simulink model "both_on_off"  (R2015b)
settings: Solver=ode23tb  StartTime=0.0  StopTime=2  RelTol=1e-3
PreLoadFcn:
  | load  power_3levelVSC.mat
  | Ts_Power=5e-6;
  | Ts_Control=100e-6;
libraries: powerlib x29, powerlib_extras x7, powerlib_meascontrol x6, simulink x3
settings Model: Creator=Pouyan  LastModifiedBy=fujitsu
settings DataIOCC: SaveFormat=Array  SignalLoggingSaveFormat=ModelDataLogs
settings OptimizationCC: ExpressionDepthLimit=2147483647
settings DebuggingCC: UnderspecifiedInitializationDetection=Classic  MergeDetectMultiDrivingBlocksExec=none  SolverPrmCheckMsg=warning  FcnCallInpInsideContextMsg=UseLocalSettings  StateNameClashWarn=warning
settings HardwareCC: ProdBitPerPointer=32  ProdLargestAtomicFloat=None  ProdIntDivRoundTo=Undefined  ProdEndianess=Unspecified  ProdWordSize=32  ProdHWDeviceType=32-bit Generic
settings GRTTargetCC: GeneratePreprocessorConditionals=Disable all  CombineOutputUpdateFcns=off  GRTInterface=on
settings ConfigComp: CovModelRefEnable=Off

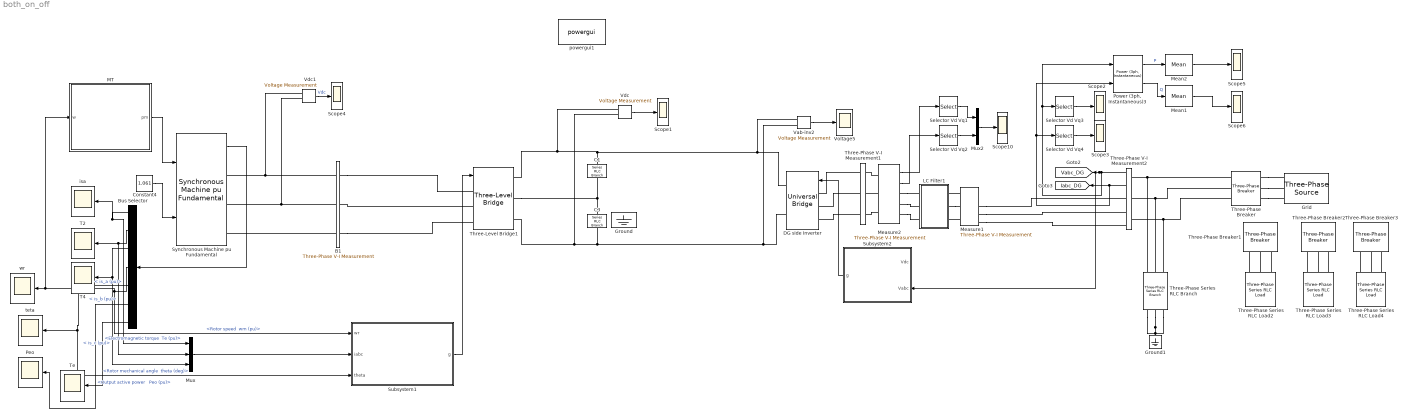
== system both_on_off ==
  B1 : powerlib/Measurements/Three-Phase V-I Measurement  VoltageMeasurement=phase-to-ground  SetLabelV=on  LabelV=Vabc_B1  Vpu=off  VpuLL=off  CurrentMeasurement=yes  SetLabelI=on  LabelI=Iabc_B1  Ipu=off  Pbase=100e6  Vbase=500e3  OutputType=Magnitude  PhasorSimulation=off  PSBequivalent=0
  Bus Selector : BusSelector  OutputSignals="Stator current. is_a (pu),Stator current. is_b (pu),Stator current. is_c (pu),Mechanical.Rotor speed  wm (pu),Mechanical.Rotor mechanical angle  theta (deg),Output active power   Peo (pu),Mechanical.Electromagnetic torque  Te (pu)"
  C1 : powerlib/Elements/Series RLC Branch  LConnTagsString=__new0  RConnTagsString=__new0  BranchType=C  Resistance=1.0  Inductance=1.0  SetiL0=off  InitialCurrent=0  Capacitance=75000e-06  Setx0=off  InitialVoltage=0  Measurements=None
  C3 : powerlib/Elements/Series RLC Branch  LConnTagsString=__new0  RConnTagsString=__new0  BranchType=C  Resistance=1.0  Inductance=1.0  SetiL0=off  InitialCurrent=0  Capacitance=75000e-06  Setx0=off  InitialVoltage=0  Measurements=None
  Constant4 : Constant  Value=1.061
  DG side Inverter : powerlib/Power Electronics/Universal Bridge  Arms=3  SnubberResistance=10000  SnubberCapacitance=inf  Device=IGBT / Diodes  Ron=1e-4  Lon=0  ForwardVoltages="[  1  1  ]"  ForwardVoltage=.8  GTOparameters=[ 10e-6 , 20e-6 ]  IGBTparameters=[ 1e-6 , 2e-6 ]  Measurements=None  Measurements_2=None  converterType=Rectifier
  Grid : powerlib/Electrical Sources/Three-Phase Source  InternalConnection=Yg  VoltagePhases=off  Voltage=400  PhaseAngle=0  Voltage_phases=[25e3 25e3 25e3]/sqrt(3)  PhaseAngles_phases=[0 -120 +120]  Frequency=50  NonIdealSource=on  SpecifyImpedance=off  Resistance=0.02  Inductance=0.3e-3  ShortCircuitLevel=100e6  BaseVoltage=25e3  XRratio=7  BusType=swing  Pref=0  Qref=0  Prefabc=[10e3, 10e3, 10e3]  Qrefabc=[0, 0, 0]  Qmin=-inf  Qmax=inf
  Ground : powerlib/Elements/Ground  LConnTagsString=a
  Ground1 : powerlib/Elements/Ground  LConnTagsString=a
  LC Filter1 : Subsystem
  MT : Subsystem
  Mean1 : powerlib_meascontrol/Measurements/Mean  Freq=50  Vinit=0  Ts=50e-6
  Mean2 : powerlib_meascontrol/Measurements/Mean  Freq=50  Vinit=0  Ts=50e-6
  Measure1 : powerlib/Measurements/Three-Phase V-I Measurement  VoltageMeasurement=phase-to-phase  SetLabelV=off  LabelV=V1  Vpu=off  VpuLL=off  CurrentMeasurement=yes  SetLabelI=off  LabelI=I1  Ipu=off  Pbase=10e3  Vbase=400  OutputType=Magnitude  PhasorSimulation=off  PSBequivalent=0
  Measure2 : powerlib/Measurements/Three-Phase V-I Measurement  VoltageMeasurement=phase-to-phase  SetLabelV=off  LabelV=V1  Vpu=off  VpuLL=on  CurrentMeasurement=yes  SetLabelI=off  LabelI=I1  Ipu=on  Pbase=30e3  Vbase=380  OutputType=Magnitude  PhasorSimulation=off  PSBequivalent=0
  Mux : Mux  Inputs=3
  Mux2 : Mux  Inputs=2
  Peo : Scope
  "Power (3ph, Instantaneous)3" : powerlib_meascontrol/Measurements/Power (3ph, Instantaneous)
  Scope{1..6,10} (7 alike) : Scope
  Selector Vd Vq{1..4} (4 alike) : Selector  InputPortWidth=3  IndexOptions=Index vector (dialog)  Indices=[1]  OutputSizes=1
  Subsystem1 : Subsystem  mask{kp=1, ki=5}
  Subsystem2 : Subsystem  mask{kp=0.0001, ki=5}
  Synchronous Machine pu Fundamental : powerlib/Machines/Synchronous Machine pu Fundamental  PresetModel=No  MechanicalLoad=Mechanical power Pm  ShowDetailedParameters=on  RotorType=Salient-pole  Units=per unit fundamental parameters  MeasurementBus=off  NominalParameters="[ 60e3  500 1600]"  Stator="[ 0.2503  0.114  0.6875  0.6875 ]"  Field="[ 1  10e15/(100*pi)]"  Dampers2=[0.0652, 0.5134, 0.0287, 0.2553, 7.765e-3, 0.9167 ]  Dampers1="[ 1.17E-02  0.182  1.97E-02  0.384 ]"  Mechanical=[ 6 0 2]  PolePairs=20  InitialConditions="[ 0  0  0  0  0  0  0  0  1 ]"  SetSaturation=off  Saturation=[0.6404,0.7127,0.8441,0.9214,0.9956,1.082,1.19,1.316,1.457;0.7,0.7698,0.8872,0.9466,0.9969,1.046,1.1,1.151,1.201]  LoadFlowParameters=[1,0,0,0,0]  TsPowergui=0  TsBlock=-1  IterativeModel=Trapezoidal non iterative  BusType=swing  Pref=0  Qref=0  Qmin=-inf  Qmax=inf  PLF=0  QLF=0
  T2 : Scope
  T4 : Scope
  Te : Scope
  Three-Level Bridge1 : powerlib/Power Electronics/Three-Level Bridge  Arms=3  SnubberResistance=100  SbubberCapacitance=1e-6  Device=IGBT / Diodes  Ron=5e-3  ForwardVoltages=[370 1]  Measurements=All voltages and currents
  Three-Phase Series RLC Branch : powerlib/Elements/Three-Phase Series RLC Branch  LConnTagsString=A|B|C  RConnTagsString=A|B|C  BranchType=R  Resistance=400^2/50000  Inductance=1e-3  Capacitance=1e-6  Measurements=None
  Three-Phase Series RLC Load2 : powerlib/Elements/Three-Phase Series RLC Load  LConnTagsString=A|B|C  Configuration=Y (grounded)  NominalVoltage=380  Vabc=[1e3 1e3 1e3]  Vabcp=[1e3 1e3 1e3]  NominalFrequency=50  UnbalancedPower=off  ActivePower=50e3  InductivePower=0  CapacitivePower=0  Pabc=[10e3 9e3 11e3]  QLabc=[100 90 110]  QCabc=[100 90 110]  Pabcp=[10e3 9e3 11e3]  QLabcp=[100 90 110]  QCabcp=[100 90 110]  Measurements=None  LoadType=constant Z
  Three-Phase Series RLC Load3 : powerlib/Elements/Three-Phase Series RLC Load  LConnTagsString=A|B|C  Configuration=Y (grounded)  NominalVoltage=380  Vabc=[1e3 1e3 1e3]  Vabcp=[1e3 1e3 1e3]  NominalFrequency=50  UnbalancedPower=off  ActivePower=15e3  InductivePower=0  CapacitivePower=0  Pabc=[10e3 9e3 11e3]  QLabc=[100 90 110]  QCabc=[100 90 110]  Pabcp=[10e3 9e3 11e3]  QLabcp=[100 90 110]  QCabcp=[100 90 110]  Measurements=None  LoadType=constant Z
  Three-Phase Series RLC Load4 : powerlib/Elements/Three-Phase Series RLC Load  LConnTagsString=A|B|C  Configuration=Y (grounded)  NominalVoltage=380  Vabc=[1e3 1e3 1e3]  Vabcp=[1e3 1e3 1e3]  NominalFrequency=50  UnbalancedPower=off  ActivePower=30e3  InductivePower=0  CapacitivePower=0  Pabc=[10e3 9e3 11e3]  QLabc=[100 90 110]  QCabc=[100 90 110]  Pabcp=[10e3 9e3 11e3]  QLabcp=[100 90 110]  QCabcp=[100 90 110]  Measurements=None  LoadType=constant Z
  Three-Phase V-I Measurement1 : powerlib/Measurements/Three-Phase V-I Measurement  VoltageMeasurement=no  SetLabelV=off  LabelV=Vabc  Vpu=on  VpuLL=off  CurrentMeasurement=no  SetLabelI=off  LabelI=Iabc  Ipu=on  Pbase=300e3  Vbase=208  OutputType=Complex  PhasorSimulation=off  PSBequivalent=0
  Three-Phase V-I Measurement2 : powerlib/Measurements/Three-Phase V-I Measurement  VoltageMeasurement=phase-to-phase  SetLabelV=off  LabelV=Vabc  Vpu=off  VpuLL=on  CurrentMeasurement=yes  SetLabelI=off  LabelI=Iabc  Ipu=on  Pbase=50e3  Vbase=400  OutputType=Complex  PhasorSimulation=off  PSBequivalent=0
  Three-Phase Breaker : powerlib/Elements/Three-Phase Breaker  InitialState=closed  SwitchA=on  SwitchB=on  SwitchC=on  SwitchTimes=[1]  External=off  BreakerResistance=0.01  SnubberResistance=1e6  SnubberCapacitance=inf  Measurements=None
  Three-Phase Breaker1 : powerlib/Elements/Three-Phase Breaker  InitialState=open  SwitchA=on  SwitchB=on  SwitchC=on  SwitchTimes=[8]  External=off  BreakerResistance=0.01  SnubberResistance=1e6  SnubberCapacitance=inf  Measurements=None
  Three-Phase Breaker2 : powerlib/Elements/Three-Phase Breaker  InitialState=closed  SwitchA=on  SwitchB=on  SwitchC=on  SwitchTimes=[6 9]  External=off  BreakerResistance=0.01  SnubberResistance=1e6  SnubberCapacitance=inf  Measurements=None
  Three-Phase Breaker3 : powerlib/Elements/Three-Phase Breaker  InitialState=open  SwitchA=on  SwitchB=on  SwitchC=on  SwitchTimes=[4]  External=off  BreakerResistance=0.01  SnubberResistance=1e6  SnubberCapacitance=inf  Measurements=None
  Vab-inv2 : powerlib/Measurements/Voltage Measurement  Tag=PoWeRsYsTeMmEaSuReMeNt  PhasorSimulation=off  OutputType=Magnitude  PSBequivalent=0
  "Vdc " : powerlib/Measurements/Voltage Measurement  Tag=PoWeRsYsTeMmEaSuReMeNt  PhasorSimulation=off  OutputType=Magnitude  PSBequivalent=0
  Vdc1 : powerlib/Measurements/Voltage Measurement  Tag=PoWeRsYsTeMmEaSuReMeNt  PhasorSimulation=off  OutputType=Magnitude  PSBequivalent=0
  Voltage5 : Scope
  isa : Scope
  powergui1 : powerlib/powergui  Priority=2  SimulationMode=Discrete  SolverType=Tustin/Backward Euler (TBE)  SampleTime=Ts_Power  frequency=60  SPID=off  DisableSnubberDevices=off  DisableRonSwitches=off  DisableVfSwitches=off  SwTol=0  DisplayEquations=off  Interpol=off  ExternalGateDelay=off  methode=off  Ts=0  FunctionMessages=off  echomessages=off  HookPort=off  EnableUseOfTLC=off  x0status=blocks  frequencyindice=0  Pbase=100e6  ErrMax=1e-4  Iterations=50  UnitsV=kV  UnitsW=MW  buscounter=0  RestoreLinks=warning  ResistiveCurrentMeasurement=off  Frange=logspace(0,3,50)  Ylog=off  Xlog=off  ShowGrid=off  save=off  variable=ZData  structure=VaIa  ZoomFFT=on  StartTime=0.2  cycles=2  DisplayStyle=1  fundamental=60  FreqAxis=off  MaxFrequency=1000  frequencyindicesteady=1  RmsSteady=2  display=off
  teta : Scope
  wr : Scope
  tag scope: Iabc_DG=global, Vabc_DG=global
  wires:
  "Vdc "/1 -> Scope1/1
  MT/1(pm) -> Synchronous Machine pu Fundamental/1
  Synchronous Machine pu Fundamental/1 -> Bus Selector/1
  Bus Selector/4 -> Subsystem1/1(wr), MT/1(w), wr/1  "<Rotor speed  wm (pu)>"
  Constant4/1 -> Synchronous Machine pu Fundamental/2
  Vdc1/1 -> Scope4/1  "Vdc"
  Bus Selector/1 -> Mux/1, isa/1  "< is_a (pu)>"
  Bus Selector/2 -> T2/1, Mux/2  "< is_b (pu)>"
  Bus Selector/3 -> Mux/3, T4/1  "< is_c (pu)>"
  Bus Selector/5 -> Subsystem1/3(theta), teta/1  "<Rotor mechanical angle  theta (deg)>"
  Mux/1 -> Subsystem1/2(iabc)
  Subsystem1/1(g) -> Three-Level Bridge1/1
  Three-Phase V-I Measurement2/1 -> Subsystem2/2(Vabc), [Vabc_DG], "Power (3ph, Instantaneous)3"/1, Selector Vd Vq3/1
  Three-Phase V-I Measurement2/2 -> "Power (3ph, Instantaneous)3"/2, Selector Vd Vq4/1, [Iabc_DG]
  Vab-inv2/1 -> Voltage5/1
  Mux2/1 -> Scope10/1
  Selector Vd Vq1/1 -> Mux2/1
  Selector Vd Vq2/1 -> Mux2/2
  Measure2/1 -> Selector Vd Vq1/1
  Measure2/2 -> Selector Vd Vq2/1
  Selector Vd Vq3/1 -> Scope2/1
  Selector Vd Vq4/1 -> Scope3/1
  "Power (3ph, Instantaneous)3"/1 -> Mean2/1  "P"
  "Power (3ph, Instantaneous)3"/2 -> Mean1/1  "Q"
  Mean2/1 -> Scope5/1
  Mean1/1 -> Scope6/1
  Subsystem2/1(g) -> DG side Inverter/1
  Bus Selector/6 -> Peo/1  "<Output active power   Peo (pu)>"
  Bus Selector/7 -> Te/1  "<Electromagnetic torque  Te (pu)>"
  connections:
  C3/LConn1 -- C1/RConn1 -- Three-Level Bridge1/RConn2
  DG side Inverter/RConn2 -- Vab-inv2/LConn2 -- Three-Level Bridge1/RConn3 -- "Vdc "/LConn2 -- C3/RConn1
  Vab-inv2/LConn1 -- DG side Inverter/RConn1 -- C1/LConn1 -- Three-Level Bridge1/RConn1 -- "Vdc "/LConn1
  B1/RConn1 -- Three-Level Bridge1/LConn1
  B1/RConn3 -- Three-Level Bridge1/LConn3
  Three-Level Bridge1/LConn2 -- B1/RConn2
  B1/LConn1 -- Vdc1/LConn1 -- Synchronous Machine pu Fundamental/RConn1
  B1/LConn2 -- Vdc1/LConn2 -- Synchronous Machine pu Fundamental/RConn2
  B1/LConn3 -- Synchronous Machine pu Fundamental/RConn3
  Three-Phase Breaker/LConn1 -- Three-Phase Series RLC Branch/LConn1 -- Three-Phase V-I Measurement2/LConn1
  Three-Phase Series RLC Branch/LConn2 -- Three-Phase Breaker/LConn2 -- Three-Phase V-I Measurement2/LConn2
  Three-Phase Series RLC Branch/LConn3 -- Three-Phase Breaker/LConn3 -- Three-Phase V-I Measurement2/LConn3
  Measure1/RConn2 -- Three-Phase V-I Measurement2/RConn2
  Measure1/RConn3 -- Three-Phase V-I Measurement2/RConn3
  Measure1/RConn1 -- Three-Phase V-I Measurement2/RConn1
  Three-Phase V-I Measurement1/RConn1 -- DG side Inverter/LConn1
  Three-Phase V-I Measurement1/RConn2 -- DG side Inverter/LConn2
  Three-Phase V-I Measurement1/RConn3 -- DG side Inverter/LConn3
  Measure1/LConn1 -- LC Filter1/RConn1
  Measure1/LConn3 -- LC Filter1/RConn3
  Measure2/LConn2 -- Three-Phase V-I Measurement1/LConn2
  Measure2/LConn1 -- Three-Phase V-I Measurement1/LConn1
  Measure2/LConn3 -- Three-Phase V-I Measurement1/LConn3
  Measure2/RConn1 -- LC Filter1/LConn1
  Measure2/RConn2 -- LC Filter1/LConn2
  Measure2/RConn3 -- LC Filter1/LConn3
  LC Filter1/RConn2 -- Measure1/LConn2
  Three-Phase Breaker/RConn1 -- Grid/RConn1
  Three-Phase Breaker/RConn2 -- Grid/RConn2
  Three-Phase Breaker/RConn3 -- Grid/RConn3
  Three-Phase Series RLC Load2/LConn1 -- Three-Phase Breaker1/RConn3
  Three-Phase Series RLC Load2/LConn2 -- Three-Phase Breaker1/RConn2
  Three-Phase Series RLC Load2/LConn3 -- Three-Phase Breaker1/RConn1
  Three-Phase Series RLC Load3/LConn1 -- Three-Phase Breaker2/RConn3
  Three-Phase Series RLC Load3/LConn2 -- Three-Phase Breaker2/RConn2
  Three-Phase Series RLC Load3/LConn3 -- Three-Phase Breaker2/RConn1
  Three-Phase Series RLC Load4/LConn1 -- Three-Phase Breaker3/RConn3
  Three-Phase Series RLC Load4/LConn2 -- Three-Phase Breaker3/RConn2
  Three-Phase Series RLC Load4/LConn3 -- Three-Phase Breaker3/RConn1
  Three-Phase Series RLC Branch/RConn1 -- Three-Phase Series RLC Branch/RConn3 -- Three-Phase Series RLC Branch/RConn2 -- Ground1/LConn1

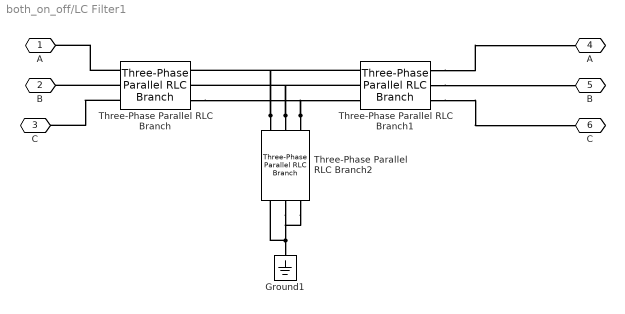
== system both_on_off/LC Filter1 ==
  Ground1 : powerlib/Elements/Ground  LConnTagsString=a
  Three-Phase Parallel RLC Branch : powerlib/Elements/Three-Phase Parallel RLC Branch  LConnTagsString=A|B|C  RConnTagsString=A|B|C  BranchType=L  Resistance=1  Inductance=5.7e-3  Capacitance=1e-6  Measurements=None
  Three-Phase Parallel RLC Branch1 : powerlib/Elements/Three-Phase Parallel RLC Branch  LConnTagsString=A|B|C  RConnTagsString=A|B|C  BranchType=R  Resistance=0.00001  Inductance=5.7e-3  Capacitance=1e-6  Measurements=None
  Three-Phase Parallel RLC Branch2 : powerlib/Elements/Three-Phase Parallel RLC Branch  LConnTagsString=A|B|C  RConnTagsString=A|B|C  BranchType=C  Resistance=1  Inductance=5.7e-3  Capacitance=1000e-6  Measurements=None
  A : PMIOPort  Port=1  Side=Left
  B : PMIOPort  Port=2  Side=Left
  C : PMIOPort  Port=3  Side=Left
  "A " : PMIOPort  Port=4  Side=Right
  "B " : PMIOPort  Port=5  Side=Right
  "C " : PMIOPort  Port=6  Side=Right
  connections:
  Ground1/LConn1 -- Three-Phase Parallel RLC Branch2/RConn2 -- Three-Phase Parallel RLC Branch2/RConn1 -- Three-Phase Parallel RLC Branch2/RConn3
  Three-Phase Parallel RLC Branch1/RConn3 -- "C "/RConn1
  Three-Phase Parallel RLC Branch1/RConn2 -- "B "/RConn1
  Three-Phase Parallel RLC Branch1/RConn1 -- "A "/RConn1
  Three-Phase Parallel RLC Branch2/LConn3 -- Three-Phase Parallel RLC Branch1/LConn3 -- Three-Phase Parallel RLC Branch/RConn3
  Three-Phase Parallel RLC Branch2/LConn2 -- Three-Phase Parallel RLC Branch/RConn2 -- Three-Phase Parallel RLC Branch1/LConn2
  Three-Phase Parallel RLC Branch2/LConn1 -- Three-Phase Parallel RLC Branch/RConn1 -- Three-Phase Parallel RLC Branch1/LConn1
  Three-Phase Parallel RLC Branch/LConn3 -- C/RConn1
  Three-Phase Parallel RLC Branch/LConn2 -- B/RConn1
  Three-Phase Parallel RLC Branch/LConn1 -- A/RConn1

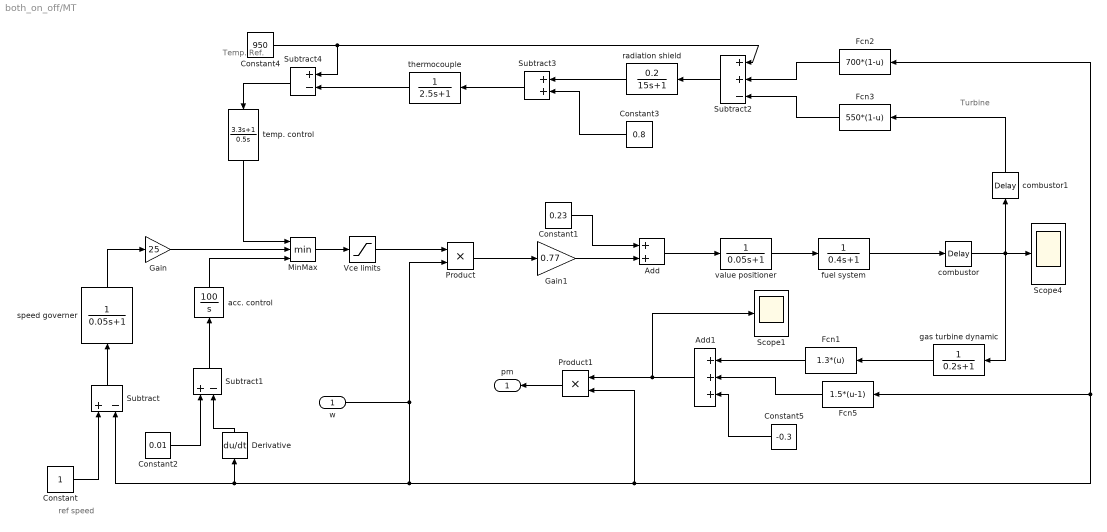
== system both_on_off/MT ==
  note: ref speed
  note: Temp.
      | Ref.
  note: Turbine
  w : Inport
  Add : Sum
  Add1 : Sum  Inputs=+++
  Constant : Constant
  Constant1 : Constant  Value=0.23
  Constant2 : Constant  Value=0.01
  Constant3 : Constant  Value=0.8
  Constant4 : Constant  Value=950
  Constant5 : Constant  Value=-0.3
  Derivative : Derivative  CoefficientInTFapproximation=0.001
  Fcn1 : Fcn  Expr=1.3*(u)
  Fcn2 : Fcn  Expr=700*(1-u)
  Fcn3 : Fcn  Expr=550*(1-u)
  Fcn5 : Fcn  Expr=1.5*(u-1)
  Gain : Gain  Gain=25
  Gain1 : Gain  Gain=0.77
  MinMax : MinMax  Inputs=3
  Product : Product  RndMeth=Zero
  Product1 : Product  RndMeth=Zero
  Scope1 : Scope
  Scope4 : Scope
  Subtract : Sum  Inputs=+-
  Subtract1 : Sum  Inputs=+-
  Subtract2 : Sum  Inputs=++-
  Subtract3 : Sum
  Subtract4 : Sum  Inputs=+-
  Vce limits : Saturate  UpperLimit=1.5  LowerLimit=-0.1
  acc. control : TransferFcn  Numerator=[0 100]  Denominator=[1 0]
  combustor : TransportDelay  DelayTime=0.01
  combustor1 : TransportDelay  DelayTime=0.04
  fuel system : TransferFcn  Denominator=[0.4 1]
  gas turbine dynamic : TransferFcn  Denominator=[0.2 1]
  radiation shield : TransferFcn  Numerator=[0.2]  Denominator=[15 1]
  speed governer : TransferFcn  Numerator=[0 1]  Denominator=[0.05 1]
  temp. control : TransferFcn  Numerator=[3.3 1]  Denominator=[0.5 0]
  thermocouple : TransferFcn  Denominator=[2.5 1]
  value positioner : TransferFcn  Denominator=[0.05 1]
  pm : Outport
  wires:
  Constant/1 -> Subtract/1
  Subtract/1 -> speed governer/1
  Vce limits/1 -> Product/1
  Product/1 -> Gain1/1
  Gain1/1 -> Add/2
  Constant1/1 -> Add/1
  Add/1 -> value positioner/1
  value positioner/1 -> fuel system/1
  fuel system/1 -> combustor/1
  combustor/1 -> gas turbine dynamic/1, combustor1/1, Scope4/1
  Add1/1 -> Scope1/1, Product1/1
  Gain/1 -> MinMax/2
  Derivative/1 -> Subtract1/2
  Constant2/1 -> Subtract1/1
  Subtract1/1 -> acc. control/1
  acc. control/1 -> MinMax/3
  MinMax/1 -> Vce limits/1
  combustor1/1 -> Fcn3/1
  Fcn3/1 -> Subtract2/3
  Fcn2/1 -> Subtract2/2
  radiation shield/1 -> Subtract3/1
  Constant3/1 -> Subtract3/2
  Subtract2/1 -> radiation shield/1
  Subtract3/1 -> thermocouple/1
  thermocouple/1 -> Subtract4/2
  Constant4/1 -> Subtract4/1, Subtract2/1
  Subtract4/1 -> temp. control/1
  temp. control/1 -> MinMax/1
  speed governer/1 -> Gain/1
  w/1 -> Product/2, Product1/2, Fcn2/1, Fcn5/1, Derivative/1, Subtract/2
  gas turbine dynamic/1 -> Fcn1/1
  Fcn1/1 -> Add1/1
  Constant5/1 -> Add1/3
  Fcn5/1 -> Add1/2
  Product1/1 -> pm/1

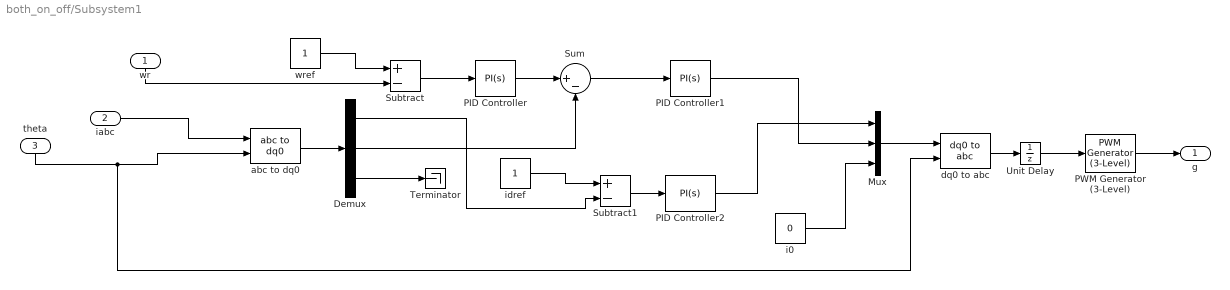
== system both_on_off/Subsystem1 ==
  wr : Inport
  iabc : Inport  Port=2
  theta : Inport  Port=3
  Demux : Demux  Outputs=3
  Mux : Mux  Inputs=3
  PID Controller : simulink/Continuous/PID Controller  Controller=PI  TimeDomain=Continuous-time  SampleTime=-1  IntegratorMethod=Forward Euler  FilterMethod=Forward Euler  Form=Parallel  UseFilter=on  ControllerParametersSource=internal  P=kp  I=ki  D=0  N=100  InitialConditionSource=internal  InitialConditionForIntegrator=0  InitialConditionForFilter=0  ExternalReset=none  LimitOutput=off  UpperSaturationLimit=inf  LowerSaturationLimit=-inf  LinearizeAsGain=on  AntiWindupMode=none  Kb=1  TrackingMode=off  Kt=1  PParamMin=[]  PParamMax=[]  IParamMin=[]  IParamMax=[]  DParamMin=[]  DParamMax=[]  NParamMin=[]  NParamMax=[]  KbParamMin=[]  KbParamMax=[]  KtParamMin=[]  KtParamMax=[]  POutMin=[]  POutMax=[]  IOutMin=[]  IOutMax=[]  DOutMin=[]  DOutMax=[]  NOutMin=[]  NOutMax=[]  KbOutMin=[]  KbOutMax=[]  KtOutMin=[]  KtOutMax=[]  IntegratorOutMin=[]  IntegratorOutMax=[]  FilterOutMin=[]  FilterOutMax=[]  SumOutMin=[]  SumOutMax=[]  SumI1OutMin=[]  SumI1OutMax=[]  SumI2OutMin=[]  SumI2OutMax=[]  SumI3OutMin=[]  SumI3OutMax=[]  SumDOutMin=[]  SumDOutMax=[]  SaturationOutMin=[]  SaturationOutMax=[]  IntegratorContinuousStateAttributes=''  IntegratorStateMustResolveToSignalObject=off  IntegratorRTWStateStorageClass=Auto  FilterContinuousStateAttributes=''  FilterStateMustResolveToSignalObject=off  FilterRTWStateStorageClass=Auto  DifferentiatorICPrevScaledInput=0  DifferentiatorOutMin=[]  DifferentiatorOutMax=[]
  PID Controller1 : simulink/Continuous/PID Controller  Controller=PI  TimeDomain=Continuous-time  SampleTime=-1  IntegratorMethod=Forward Euler  FilterMethod=Forward Euler  Form=Parallel  UseFilter=on  ControllerParametersSource=internal  P=kp  I=ki  D=0  N=100  InitialConditionSource=internal  InitialConditionForIntegrator=0  InitialConditionForFilter=0  ExternalReset=none  LimitOutput=off  UpperSaturationLimit=inf  LowerSaturationLimit=-inf  LinearizeAsGain=on  AntiWindupMode=none  Kb=1  TrackingMode=off  Kt=1  PParamMin=[]  PParamMax=[]  IParamMin=[]  IParamMax=[]  DParamMin=[]  DParamMax=[]  NParamMin=[]  NParamMax=[]  KbParamMin=[]  KbParamMax=[]  KtParamMin=[]  KtParamMax=[]  POutMin=[]  POutMax=[]  IOutMin=[]  IOutMax=[]  DOutMin=[]  DOutMax=[]  NOutMin=[]  NOutMax=[]  KbOutMin=[]  KbOutMax=[]  KtOutMin=[]  KtOutMax=[]  IntegratorOutMin=[]  IntegratorOutMax=[]  FilterOutMin=[]  FilterOutMax=[]  SumOutMin=[]  SumOutMax=[]  SumI1OutMin=[]  SumI1OutMax=[]  SumI2OutMin=[]  SumI2OutMax=[]  SumI3OutMin=[]  SumI3OutMax=[]  SumDOutMin=[]  SumDOutMax=[]  SaturationOutMin=[]  SaturationOutMax=[]  IntegratorContinuousStateAttributes=''  IntegratorStateMustResolveToSignalObject=off  IntegratorRTWStateStorageClass=Auto  FilterContinuousStateAttributes=''  FilterStateMustResolveToSignalObject=off  FilterRTWStateStorageClass=Auto  DifferentiatorICPrevScaledInput=0  DifferentiatorOutMin=[]  DifferentiatorOutMax=[]
  PID Controller2 : simulink/Continuous/PID Controller  Controller=PI  TimeDomain=Continuous-time  SampleTime=-1  IntegratorMethod=Forward Euler  FilterMethod=Forward Euler  Form=Parallel  UseFilter=on  ControllerParametersSource=internal  P=kp  I=ki  D=0  N=100  InitialConditionSource=internal  InitialConditionForIntegrator=0  InitialConditionForFilter=0  ExternalReset=none  LimitOutput=off  UpperSaturationLimit=inf  LowerSaturationLimit=-inf  LinearizeAsGain=on  AntiWindupMode=none  Kb=1  TrackingMode=off  Kt=1  PParamMin=[]  PParamMax=[]  IParamMin=[]  IParamMax=[]  DParamMin=[]  DParamMax=[]  NParamMin=[]  NParamMax=[]  KbParamMin=[]  KbParamMax=[]  KtParamMin=[]  KtParamMax=[]  POutMin=[]  POutMax=[]  IOutMin=[]  IOutMax=[]  DOutMin=[]  DOutMax=[]  NOutMin=[]  NOutMax=[]  KbOutMin=[]  KbOutMax=[]  KtOutMin=[]  KtOutMax=[]  IntegratorOutMin=[]  IntegratorOutMax=[]  FilterOutMin=[]  FilterOutMax=[]  SumOutMin=[]  SumOutMax=[]  SumI1OutMin=[]  SumI1OutMax=[]  SumI2OutMin=[]  SumI2OutMax=[]  SumI3OutMin=[]  SumI3OutMax=[]  SumDOutMin=[]  SumDOutMax=[]  SaturationOutMin=[]  SaturationOutMax=[]  IntegratorContinuousStateAttributes=''  IntegratorStateMustResolveToSignalObject=off  IntegratorRTWStateStorageClass=Auto  FilterContinuousStateAttributes=''  FilterStateMustResolveToSignalObject=off  FilterRTWStateStorageClass=Auto  DifferentiatorICPrevScaledInput=0  DifferentiatorOutMin=[]  DifferentiatorOutMax=[]
  PWM Generator (3-Level) : powerlib_meascontrol/Pulse & Signal Generators/PWM Generator (3-Level)  ModulatorType=Three-phase bridge (12 pulses)  ModulatorMode=Unsynchronized  nF=27  Fc=20e3  ModulatingSignals=off  m=0.8  Freq=60  Phase=0  Ts=Ts_Power
  Subtract : Sum  Inputs=+-
  Subtract1 : Sum  Inputs=+-
  Sum : Sum  Inputs=|+-
  Terminator : Terminator
  Unit Delay : UnitDelay  SampleTime=Ts_Control
  abc to dq0 : powerlib_meascontrol/Transformations/abc to dq0  Alignment=90 degrees behind phase A axis
  dq0 to abc : powerlib_meascontrol/Transformations/dq0 to abc  Alignment=90 degrees behind phase A axis
  i0 : Constant  Value=0
  idref : Constant
  wref : Constant
  g : Outport
  wires:
  Sum/1 -> PID Controller1/1
  Subtract/1 -> PID Controller/1
  wref/1 -> Subtract/1
  iabc/1 -> abc to dq0/1
  Demux/2 -> Sum/2
  Subtract1/1 -> PID Controller2/1
  theta/1 -> dq0 to abc/2, abc to dq0/2
  wr/1 -> Subtract/2
  Demux/1 -> Subtract1/2
  idref/1 -> Subtract1/1
  abc to dq0/1 -> Demux/1
  PID Controller/1 -> Sum/1
  Demux/3 -> Terminator/1
  i0/1 -> Mux/3
  PID Controller1/1 -> Mux/2
  PID Controller2/1 -> Mux/1
  Mux/1 -> dq0 to abc/1
  dq0 to abc/1 -> Unit Delay/1
  PWM Generator (3-Level)/1 -> g/1
  Unit Delay/1 -> PWM Generator (3-Level)/1

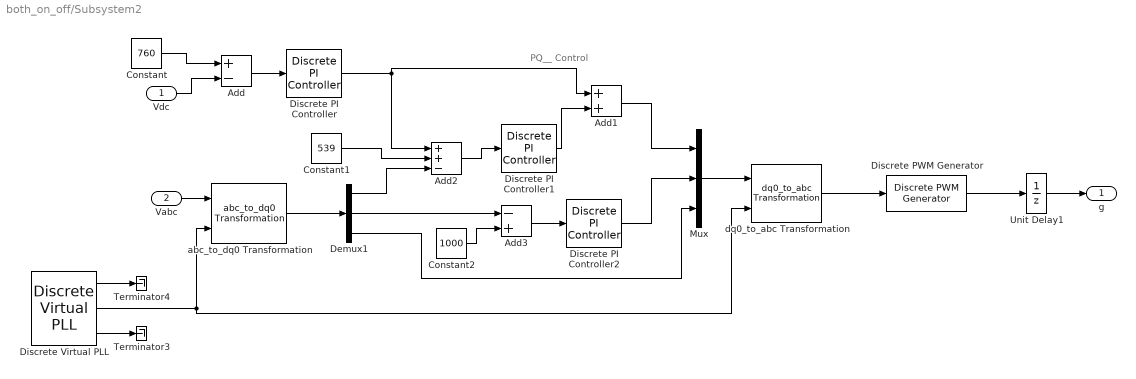
== system both_on_off/Subsystem2 ==
  note: PQ__ Control
  Vdc : Inport
  Vabc : Inport  Port=2
  Add : Sum  Inputs=+-
  Add1 : Sum
  Add2 : Sum  Inputs=++-
  Add3 : Sum  Inputs=-+
  Constant : Constant  Value=760
  Constant1 : Constant  Value=539
  Constant2 : Constant  Value=1000
  Demux1 : Demux  Outputs=3
  Discrete PI Controller : powerlib_extras/Discrete  Control Blocks/Discrete PI Controller  Kp=kp  Ki=ki  Par_Limits=[1e6 -1e6]  Init=0  Ts=50e-6
  Discrete PI Controller1 : powerlib_extras/Discrete  Control Blocks/Discrete PI Controller  Kp=kp  Ki=ki  Par_Limits=[1e6 -1e6]  Init=0  Ts=50e-6
  Discrete PI Controller2 : powerlib_extras/Discrete  Control Blocks/Discrete PI Controller  Kp=kp  Ki=ki  Par_Limits=[1e6 -1e6]  Init=0  Ts=50e-6
  Discrete PWM Generator : powerlib_extras/Discrete  Control Blocks/Discrete PWM Generator  GeneratorMode="3-arm  bridge (6 pulses)"  Fc=8e3  Ts=2e-6  Internal=off  mIndex=0.4  Freq=60  Phase=0
  Discrete Virtual PLL : powerlib_extras/Discrete  Control Blocks/Discrete Virtual PLL  Freq=50  Phase=0  Ts=50e-6
  Mux : Mux  Inputs=3
  Terminator3 : Terminator
  Terminator4 : Terminator
  Unit Delay1 : UnitDelay  SampleTime=2e-6
  abc_to_dq0 Transformation : powerlib_extras/Measurements/abc_to_dq0 Transformation
  dq0_to_abc Transformation : powerlib_extras/Measurements/dq0_to_abc Transformation
  g : Outport
  wires:
  Constant/1 -> Add/1
  Vdc/1 -> Add/2
  Add/1 -> Discrete PI Controller/1
  Discrete PI Controller/1 -> Add1/1, Add2/1
  Constant1/1 -> Add2/2
  Add2/1 -> Discrete PI Controller1/1
  Discrete PI Controller1/1 -> Add1/2
  Add1/1 -> Mux/1
  Vabc/1 -> abc_to_dq0 Transformation/1
  abc_to_dq0 Transformation/1 -> Demux1/1
  Demux1/1 -> Add2/3
  Demux1/2 -> Add3/1
  Constant2/1 -> Add3/2
  Add3/1 -> Discrete PI Controller2/1
  Discrete PI Controller2/1 -> Mux/2
  Demux1/3 -> Mux/3
  Discrete Virtual PLL/1 -> Terminator4/1
  Discrete Virtual PLL/3 -> Terminator3/1
  Discrete Virtual PLL/2 -> abc_to_dq0 Transformation/2, dq0_to_abc Transformation/2
  Mux/1 -> dq0_to_abc Transformation/1
  Discrete PWM Generator/1 -> Unit Delay1/1
  dq0_to_abc Transformation/1 -> Discrete PWM Generator/1
  Unit Delay1/1 -> g/1
